simulink model "testPressureCells"  (R2017b)
settings: Solver=FixedStepDiscrete  StartTime=0.0  StopTime=inf  FixedStep=0.001  RelTol=1e-3
libraries: dspnetwork x2
settings Model: Creator=exo-hand  LastModifiedBy=exo-hand

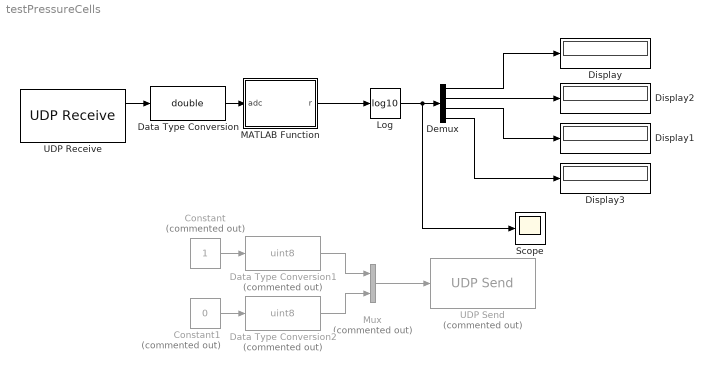
== system testPressureCells ==
  Constant : Constant  Commented=on
  Constant1 : Constant  Commented=on  Value=0
  Data Type Conversion : DataTypeConversion  OutDataTypeStr=double
  Data Type Conversion1 : DataTypeConversion  Commented=on  OutDataTypeStr=uint8
  Data Type Conversion2 : DataTypeConversion  Commented=on  OutDataTypeStr=uint8
  Demux : Demux
  Display{,1..3} (4 alike) : Display
  Log : Math  Operator=log10  SaturateOnIntegerOverflow=on
  MATLAB Function : MATLAB Function  TreatAsAtomicUnit=on
  Mux : Mux  Commented=on  Inputs=2
  Scope : Scope
  UDP Receive : dspnetwork/UDP Receive  localURL='0.0.0.0'  localPort=8000  remoteURL='10.25.4.40'  remotePort=-1  recvBufferSize=64  dims=4  signalDatatype=uint16  isVarSize=off  showBlockingTime=off  blockingTime=0  sampletime=0.001  blockPlatform=[]
      settings: SourceProductName=DSP System Toolbox  SourceProductBaseCode=DS
  UDP Send : dspnetwork/UDP Send  Commented=on  remoteURL='10.25.4.40'  remotePort=6000  localURL='0.0.0.0'  localPortSource=Automatically determine  localPort=-1  sampletime=-1  blockPlatform=[]  separateLengthPort=0
      settings: SourceProductName=DSP System Toolbox  SourceProductBaseCode=DS
  wires:
  UDP Receive/1 -> Data Type Conversion/1
  Data Type Conversion/1 -> MATLAB Function/1(adc)
  MATLAB Function/1(r) -> Log/1
  Log/1 -> Scope/1, Demux/1
  Constant/1 -> Data Type Conversion1/1
  Mux/1 -> UDP Send/1
  Data Type Conversion1/1 -> Mux/1
  Constant1/1 -> Data Type Conversion2/1
  Data Type Conversion2/1 -> Mux/2
  Demux/1 -> Display/1
  Demux/2 -> Display2/1
  Demux/3 -> Display1/1
  Demux/4 -> Display3/1

== matlab function testPressureCells/MATLAB Function ==
  data: adc input; r output
function r = fcn(adc)
%% Output resistance is expressed in Ohm
r = 1000*(4096-adc)./adc;
